simulink model "PID"  (R2023a)
settings: Solver=VariableStepAuto  StartTime=0.0  StopTime=10.0  RelTol=1e-3
settings Model: Creator=zhasi  LastModifiedBy=zhasi

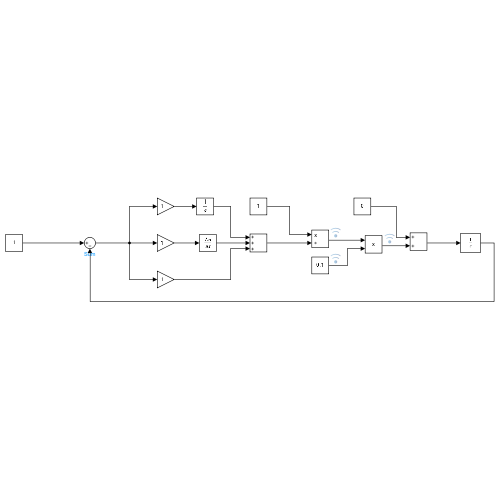
[thumbnail: Simulink's stored preview of the top-level diagram]
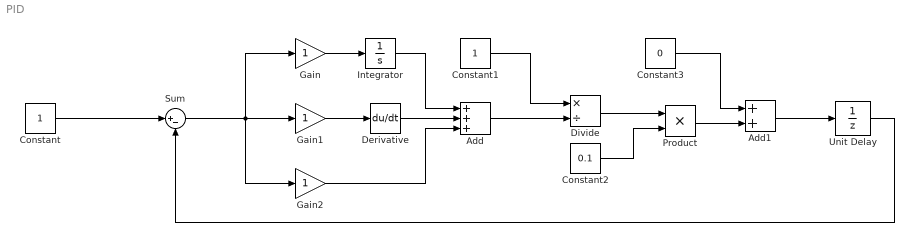
== system PID ==
  Add : Sum  Inputs=+++
  Add1 : Sum
  Constant : Constant
  Constant1 : Constant
  Constant2 : Constant  Value=0.1
  Constant3 : Constant  Value=0
  Derivative : Derivative
  Divide : Product  Inputs=*/
  Gain : Gain
  Gain1 : Gain
  Gain2 : Gain
  Integrator : Integrator
  Product : Product
  Sum : Sum  Inputs=|+-
  Unit Delay : UnitDelay  SampleTime=-1  HasFrameUpgradeWarning=on
  wires:
  Gain/1 -> Integrator/1
  Gain1/1 -> Derivative/1
  Gain2/1 -> Add/3
  Derivative/1 -> Add/2
  Integrator/1 -> Add/1
  Sum/1 -> Gain/1, Gain1/1, Gain2/1
  Constant/1 -> Sum/1
  Add/1 -> Divide/2
  Constant1/1 -> Divide/1
  Divide/1 -> Product/1
  Constant2/1 -> Product/2
  Product/1 -> Add1/2
  Constant3/1 -> Add1/1
  Add1/1 -> Unit Delay/1
  Unit Delay/1 -> Sum/2
